simulink model "simulation_sufc_new"  (R2015a)
settings: Solver=ode45  StartTime=0.0  StopTime=6.5  RelTol=1e-3
libraries: simulink x1
settings Model: Creator=Παναγιώτης Κυριάκης  LastModifiedBy=Παναγιώτης Κυριάκης

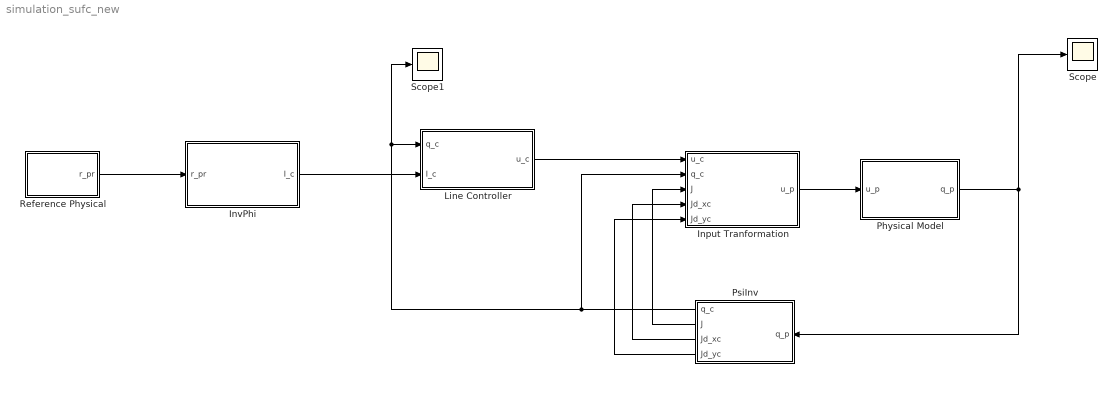
== system simulation_sufc_new ==
  "Input Tranformation " : MATLAB Function  TreatAsAtomicUnit=on
  "InvPhi " : MATLAB Function  TreatAsAtomicUnit=on
  Line Controller : MATLAB Function  TreatAsAtomicUnit=on
  Physical Model : Subsystem
  PsiInv : MATLAB Function  TreatAsAtomicUnit=on
  Reference Physical : Subsystem
  Scope : Scope
      settings: YMin=-25000  YMax=550000  SaveName=qp
  Scope1 : Scope
      settings: YMin=0  YMax=5.5  SaveName=qc
  wires:
  PsiInv/1(q_c) -> Scope1/1, Line Controller/1(q_c), "Input Tranformation "/2(q_c)
  Line Controller/1(u_c) -> "Input Tranformation "/1(u_c)
  "Input Tranformation "/1(u_p) -> Physical Model/1(u_p)
  Physical Model/1(q_p) -> Scope/1, PsiInv/1(q_p)
  Reference Physical/1(r_pr) -> "InvPhi "/1(r_pr)
  "InvPhi "/1(I_c) -> Line Controller/2(I_c)
  PsiInv/2(J) -> "Input Tranformation "/3(J)
  PsiInv/3(Jd_xc) -> "Input Tranformation "/4(Jd_xc)
  PsiInv/4(Jd_yc) -> "Input Tranformation "/5(Jd_yc)

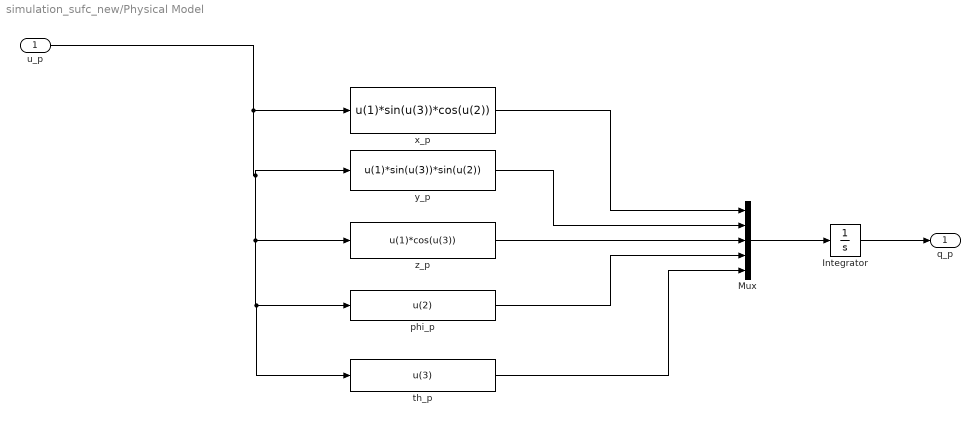
== system simulation_sufc_new/Physical Model ==
  u_p : Inport
  Integrator : Integrator  InitialCondition=[-0.5 10 2.5 pi/1.5 -pi/15]'  UpperSaturationLimit=1000  LowerSaturationLimit=-1000
  Mux : Mux  Inputs=5
  phi_p : Fcn  Expr=u(2)
  th_p : Fcn  Expr=u(3)
  "x_p " : Fcn  Expr=u(1)*sin(u(3))*cos(u(2))
  y_p : Fcn  Expr=u(1)*sin(u(3))*sin(u(2))
  z_p : Fcn  Expr=u(1)*cos(u(3))
  q_p : Outport
  wires:
  y_p/1 -> Mux/2
  z_p/1 -> Mux/3
  th_p/1 -> Mux/5
  Integrator/1 -> q_p/1
  "x_p "/1 -> Mux/1
  phi_p/1 -> Mux/4
  Mux/1 -> Integrator/1
  u_p/1 -> th_p/1, phi_p/1, z_p/1, y_p/1, "x_p "/1

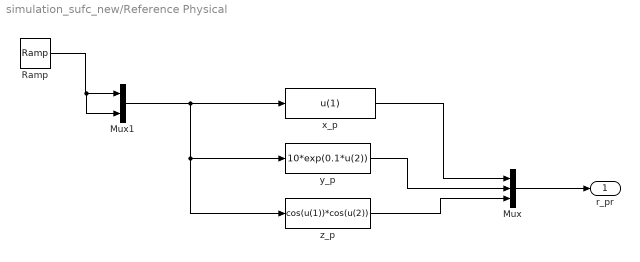
== system simulation_sufc_new/Reference Physical ==
  Mux : Mux  Inputs=3
  Mux1 : Mux  Inputs=2
  Ramp : simulink/Sources/Ramp  slope=1  start=0  X0=0
  x_p : Fcn  Expr=u(1)
  y_p : Fcn  Expr=10*exp(0.1*u(2))
  z_p : Fcn  Expr=cos(u(1))*cos(u(2))
  r_pr : Outport
  wires:
  y_p/1 -> Mux/2
  z_p/1 -> Mux/3
  x_p/1 -> Mux/1
  Mux/1 -> r_pr/1
  Ramp/1 -> Mux1/2, Mux1/1
  Mux1/1 -> z_p/1, y_p/1, x_p/1

== matlab function simulation_sufc_new/PsiInv ==
  data: q_p input; q_c output; J output; Jd_xc output; Jd_yc output
function [q_c,J,Jd_xc,Jd_yc]  = PsiInv(q_p)

    % Find canonical cordinates
    x_c = q_p(1);
    y_c = 10*log(q_p(2)/10);
    r_c = zeros(3,1);
    r_c(1,1) = x_c;
    r_c(2,1) = y_c;
    r_c(3,1) = q_p(3)-cos(x_c)*cos(y_c);
    
    
    % Find Jacobian and its derivatices
    J = [1 0 0; 0 exp(0.1*y_c) 0; -sin(x_c)*cos(y_c) -cos(x_c)*sin(y_c) 1];
    Jd_xc = [0 0 0; 0 0 0; -cos(x_c)*cos(y_c) sin(x_c)*sin(y_c) 0];
    Jd_yc = [0 0 0; 0 0.1*exp(0.1*y_c) 0; sin(x_c)*sin(y_c) -cos(x_c)*cos(y_c) 1];
    
    % Get physical angles and their unit vector
    th_p = q_p(5);
    phi_p = q_p(4);
    cp = [sin(th_p)*cos(phi_p);sin(th_p)*sin(phi_p);cos(th_p)];

    % Find canonical phi, th   
    cc = inv(J)*cp/norm(inv(J)*cp);    
    phi_c = atan2(cc(2),cc(1));
    th_c = acos(cc(3));
    
    % Canonical space-state vector
    q_c =[r_c;phi_c;th_c];   
    %q_c = q_p;
end

== matlab function simulation_sufc_new/Input Tranformation  ==
  data: u_c input; q_c input; J input; u_p output; Jd_xc input; Jd_yc input
function u_p = M(u_c,q_c,J,Jd_xc,Jd_yc)
    
    % Initialization
    C = zeros(2,3);
    D = eye(2);
    M = eye(3);
    
    % Construct needed elements of Cartesian tensor
    e12=[1 0 0]'*[0 1 0];
    e21=[0 1 0]'*[1 0 0];
    e33=[0 0 1]'*[0 0 1];
    
    % Get canonical angles
    th_c = q_c(5);
    phi_c = q_c(4);    
    
    % Construct the vector cc and its derivatives
    cc = [sin(th_c)*cos(phi_c);sin(th_c)*sin(phi_c);cos(th_c)];
    cc_phi_c = [-sin(th_c)*sin(phi_c);sin(th_c)*cos(phi_c);0];
    cc_th_c = [cos(th_c)*cos(phi_c);cos(th_c)*sin(phi_c);-sin(th_c)];
    
    % Find the length ratio
    gamma = sqrt(cc'*(J')*J*cc);
    % Find the coefficients appearing in C,D
    Aphi = (cc')*(J')*(e12-e21)/(gamma^2-(cc')*(J')*e33*J*cc);
    Ath = -gamma*[0 0 1]/sqrt(gamma^2-(cc')*(J')*e33*J*cc);

    % Find C
    C(1,1) = Aphi*Jd_xc*cc;
    C(2,1) = Ath*(2*(gamma^2)*Jd_xc-(cc')*((Jd_xc')*J+(J')*Jd_xc)*cc*J)*cc/(2*gamma^3);
    C(1,2) = Aphi*Jd_yc*cc;
    C(2,2) = Ath*(2*(gamma^2)*Jd_yc-(cc')*((Jd_yc')*J+(J')*Jd_yc)*cc*J)*cc/(2*gamma^3);

    % Find D
    D(1,1) = Aphi*J*cc_phi_c;
    D(1,2) = Aphi*J*cc_th_c;
    D(2,1) = Ath*J*(cc_phi_c*(cc')-cc*(cc_phi_c'))*(J')*J*cc/gamma^3;
    D(2,2) = Ath*J*(cc_th_c*(cc')-cc*(cc_th_c'))*(J')*J*cc/gamma^3;

    % Find M
    
    M(1,1) = gamma;
    M(2:3,1) = C*cc;
    M(2:3,2:3) = D;

    % Transform the control
    u_p = M*u_c;
    
    phi_dot_max = 5;
    th_dot_max=2.2;
    if(u_p(2)>phi_dot_max) 
        u_p(2)=phi_dot_max;
    end
    if(u_p(2)<-phi_dot_max) 
        u_p(2)=-phi_dot_max;
    end
    if(u_p(3)>th_dot_max) 
        u_p(3)=th_dot_max;
    end
    if(u_p(3)<-th_dot_max) 
        u_p(3)=-th_dot_max;
    end

 end

== matlab function simulation_sufc_new/Line Controller ==
  data: q_c input; u_c output; I_c input
function u_c = LineCon(q_c,I_c)

    K1 = -1000*[5 0 0; 0 5 0;0 0 10];     
    K2 = -320*[1 0 0; 0 1 0;0 0 0];    
    
    r_c = [q_c(1); q_c(2); q_c(3)];
    
    null_Ic= null([1 1 0]);
    nlat = null_Ic(:,1);
    nlon = null_Ic(:,2);
        
    v = K1*(nlon*nlon'+nlat*nlat')*(r_c - [0;0;1]) + K2*(cross(nlon,nlat));

    v=1.7*v/norm(v);
    
    u_c = [norm(v); atan2(v(2),v(1));acos(v(3)/norm(v))];    

end

== matlab function simulation_sufc_new/InvPhi  ==
  data: I_c output; r_pr input
function I_c  = Init(r_pr)

    x_c = r_pr(1);
    y_c = 10*log(r_pr(2)/10);
    I_c = zeros(3,1);
    I_c(1,1) = x_c;
    I_c(2,1) = y_c;
    I_c(3,1) = r_pr(3)-cos(x_c)*cos(y_c);   
end
